simulink model "modele_non_lineaire"  (R2021a)
settings: Solver=VariableStepAuto  StartTime=0.0  StopTime=tfin  RelTol=1e-3
values from neighbouring files (symbols this model uses):
  ae0 = 1.339300    (= 1.3393)    [bancEssaiConstantes.m]
  ae1 = 3.57e+02    (= 357)    [bancEssaiConstantes.m]
  ae2 = 50.13    [bancEssaiConstantes.m]
  ae3 = 7.69e+05    (= 769000)    [bancEssaiConstantes.m]
  as0 = 0.0587    [bancEssaiConstantes.m]
  as1 = 22.606    [bancEssaiConstantes.m]
  as2 = 7.4466e+02    (= 744.66)    [bancEssaiConstantes.m]
  as3 = 2.458e+05    (= 245800)    [bancEssaiConstantes.m]
  be1 = 13.029359254409743    (= 13.0293592544)    [bancEssaiConstantes.m]
  g = 9.81    [bancEssaiConstantes.m]
  Jx = 1169e-06    (= 0.001169)    [bancEssaiConstantes.m]
  Jy = Jx    (= 0.001169)    [bancEssaiConstantes.m]
  LA = LL    (= 0.115)    [bancEssaiConstantes.m]
  LB = LL    (= 0.115)    [bancEssaiConstantes.m]
  LC = LL    (= 0.115)    [bancEssaiConstantes.m]
  mP = 425e-03    (= 0.425)    [bancEssaiConstantes.m]
  mSeff = mS+JS/rS^2    (= 0.0112)    [bancEssaiConstantes.m]
  mSg = mS*g    (= 0.07848)    [bancEssaiConstantes.m]
  RA = RR    (= 3.6)    [bancEssaiConstantes.m]
  RB = RR    (= 3.6)    [bancEssaiConstantes.m]
  RC = RR    (= 3.6)    [bancEssaiConstantes.m]
  XA = +rABC    (= 0.0952)    [bancEssaiConstantes.m]
  XB = -rABC*sind(30)    [bancEssaiConstantes.m]
  XC = -rABC*sind(30)    [bancEssaiConstantes.m]
  XD = +rDEF*sind(30)    [bancEssaiConstantes.m]
  XE = -rDEF    (= -0.08)    [bancEssaiConstantes.m]
  XF = +rDEF*sind(30)    [bancEssaiConstantes.m]
  YA = 0.0    (= 0)    [bancEssaiConstantes.m]
  YB = +rABC*cosd(30)    [bancEssaiConstantes.m]
  YC = -rABC*cosd(30)    [bancEssaiConstantes.m]
  YD = +rDEF*cosd(30)    [bancEssaiConstantes.m]
  YE = 0.0    (= 0)    [bancEssaiConstantes.m]
  YF = -rDEF*cosd(30)    [bancEssaiConstantes.m]
settings Model: Creator=royv2608  LastModifiedBy=User
settings SolverCC: AlgebraicLoopSolver=LineSearch

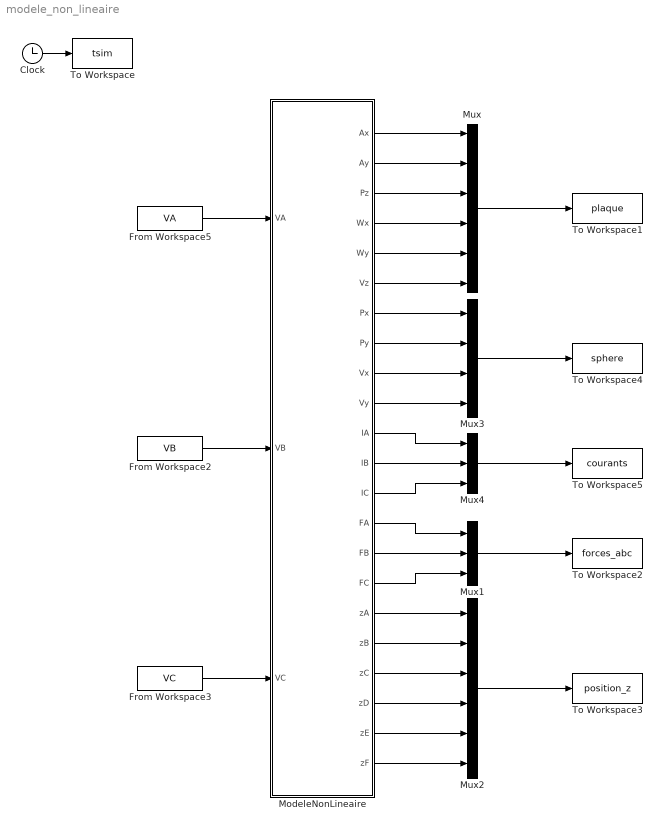
== system modele_non_lineaire ==
  Clock : Clock
  From Workspace2 : FromWorkspace  VariableName=VB  Interpolate=off  OutputAfterFinalValue=Holding final value
  From Workspace3 : FromWorkspace  VariableName=VC  Interpolate=off  OutputAfterFinalValue=Holding final value
  From Workspace5 : FromWorkspace  VariableName=VA  Interpolate=off  OutputAfterFinalValue=Holding final value
  ModeleNonLineaire : Subsystem
  Mux : Mux  Inputs=6
  Mux1 : Mux  Inputs=3
  Mux2 : Mux  Inputs=6
  Mux3 : Mux
  Mux4 : Mux  Inputs=3
  To Workspace : ToWorkspace  VariableName=tsim  SampleTime=-1
  To Workspace1 : ToWorkspace  VariableName=plaque  SampleTime=-1
  To Workspace2 : ToWorkspace  VariableName=forces_abc  SampleTime=-1
  To Workspace3 : ToWorkspace  VariableName=position_z  SampleTime=-1
  To Workspace4 : ToWorkspace  VariableName=sphere  SampleTime=-1
  To Workspace5 : ToWorkspace  VariableName=courants  SampleTime=-1
  wires:
  Clock/1 -> To Workspace/1
  Mux/1 -> To Workspace1/1
  From Workspace5/1 -> ModeleNonLineaire/1(VA)
  From Workspace3/1 -> ModeleNonLineaire/3(VC)
  ModeleNonLineaire/1(Ax) -> Mux/1
  ModeleNonLineaire/2(Ay) -> Mux/2
  ModeleNonLineaire/3(Pz) -> Mux/3
  ModeleNonLineaire/4(Wx) -> Mux/4
  ModeleNonLineaire/5(Wy) -> Mux/5
  ModeleNonLineaire/6(Vz) -> Mux/6
  ModeleNonLineaire/11(IA) -> Mux4/1
  ModeleNonLineaire/12(IB) -> Mux4/2
  ModeleNonLineaire/13(IC) -> Mux4/3
  ModeleNonLineaire/14(FA) -> Mux1/1
  ModeleNonLineaire/15(FB) -> Mux1/2
  ModeleNonLineaire/16(FC) -> Mux1/3
  Mux1/1 -> To Workspace2/1
  ModeleNonLineaire/17(zA) -> Mux2/1
  ModeleNonLineaire/19(zC) -> Mux2/3
  ModeleNonLineaire/18(zB) -> Mux2/2
  Mux2/1 -> To Workspace3/1
  From Workspace2/1 -> ModeleNonLineaire/2(VB)
  ModeleNonLineaire/20(zD) -> Mux2/4
  ModeleNonLineaire/21(zE) -> Mux2/5
  ModeleNonLineaire/22(zF) -> Mux2/6
  Mux3/1 -> To Workspace4/1
  ModeleNonLineaire/7(Px) -> Mux3/1
  ModeleNonLineaire/8(Py) -> Mux3/2
  ModeleNonLineaire/9(Vx) -> Mux3/3
  ModeleNonLineaire/10(Vy) -> Mux3/4
  Mux4/1 -> To Workspace5/1

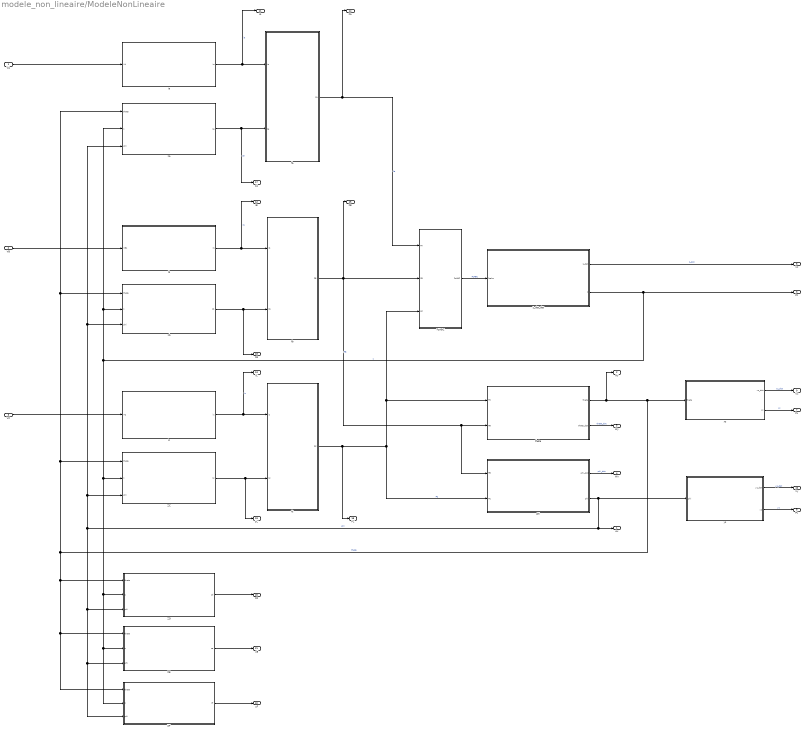
== system modele_non_lineaire/ModeleNonLineaire ==
  VA : Inport
  VB : Inport  Port=2
  VC : Inport  Port=3
  FzABC : Subsystem
  ZC : Subsystem
  ZD : Subsystem
  ZE : Subsystem
  ZF : Subsystem
  fa : Subsystem
  fb : Subsystem
  fc : Subsystem
  ia : Subsystem
  ib : Subsystem
  ic : Subsystem
  phi : Subsystem
  theta : Subsystem
  xs : Subsystem
  ys : Subsystem
  z_dot_dot : Subsystem
  za : Subsystem
  zb : Subsystem
  Ax : Outport
  Ay : Outport  Port=2
  Pz : Outport  Port=3
  Wx : Outport  Port=4
  Wy : Outport  Port=5
  Vz : Outport  Port=6
  Px : Outport  Port=7
  Py : Outport  Port=8
  Vx : Outport  Port=9
  Vy : Outport  Port=10
  IA : Outport  Port=11
  IB : Outport  Port=12
  IC : Outport  Port=13
  FA : Outport  Port=14
  FB : Outport  Port=15
  FC : Outport  Port=16
  zA : Outport  Port=17
  zB : Outport  Port=18
  zC : Outport  Port=19
  zD : Outport  Port=20
  zE : Outport  Port=21
  zF : Outport  Port=22
  wires:
  ia/1(ia) -> fa/1(ia), IA/1  "ia"
  ic/1(ic) -> IC/1, fc/1(ic)  "ic"
  phi/2(phi) -> ys/1(phi), Ax/1, za/3(phi), zb/3(phi), ZC/3(phi), ZD/3(phi), ZF/3(phi), ZE/3(phi)  "phi"
  theta/1(theta) -> xs/1(theta), ZD/1(theta), ZF/1(theta), ZE/1(theta), za/1(theta), zb/1(theta), ZC/1(theta), Ay/1  "theta"
  fa/1(FA) -> FzABC/1(FA), FA/1  "fa"
  fb/1(FB) -> FzABC/2(FB), phi/1(FB), theta/2(FB), FB/1  "FB"
  fc/1(FC) -> FC/1, phi/2(FC), FzABC/3(FC), theta/1(FC)  "FC"
  ZC/1(zc) -> zC/1, fc/2(zc)
  zb/1(zb) -> zB/1, fb/2(zb)
  ib/1(ib) -> fb/1(ib), IB/1  "ib"
  FzABC/1(FzABC) -> z_dot_dot/1(fzabc)  "FzABC"
  za/1(za) -> zA/1, fa/2(za)  "za"
  theta/2(theta_dot) -> Wy/1  "theta_dot"
  xs/1(xs_dot) -> Vx/1  "xs_dot"
  z_dot_dot/2(z) -> za/2(z), zb/2(z), ZD/2(z), ZF/2(z), ZE/2(z), ZC/2(z), Pz/1  "z"
  phi/1(phi_dot) -> Wx/1  "phi_dot"
  ys/2(ys) -> Py/1  "ys"
  VB/1 -> ib/1(VB1)
  z_dot_dot/1(z_dot) -> Vz/1  "z_dot"
  xs/2(xs) -> Px/1  "xs"
  ys/1(ys_dot) -> Vy/1  "ys_dot"
  VA/1 -> ia/1(VA)
  VC/1 -> ic/1(VC)
  ZD/1(zd) -> zD/1
  ZF/1(zf) -> zF/1
  ZE/1(ze) -> zE/1

== system modele_non_lineaire/ModeleNonLineaire/FzABC ==
  FA : Inport
  FB : Inport  Port=2
  FC : Inport  Port=3
  Sum of Elements : Sum  Inputs=---  CollapseDim=3
  FzABC : Outport
  wires:
  FC/1 -> Sum of Elements/3
  Sum of Elements/1 -> FzABC/1  "FzABC"
  FA/1 -> Sum of Elements/1
  FB/1 -> Sum of Elements/2

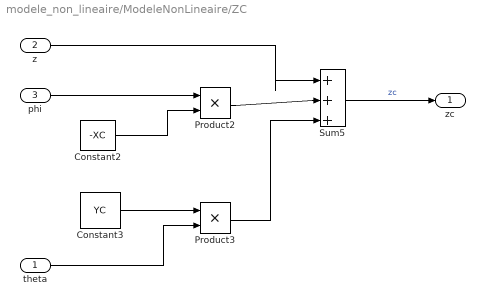
== system modele_non_lineaire/ModeleNonLineaire/ZC ==
  theta : Inport
  z : Inport  Port=2
  phi : Inport  Port=3
  Constant2 : Constant  Value=-XC
  Constant3 : Constant  Value=YC
  Product2 : Product
  Product3 : Product
  Sum5 : Sum  Inputs=|+++
  zc : Outport
  wires:
  Constant2/1 -> Product2/2
  z/1 -> Sum5/1
  theta/1 -> Product3/2
  Constant3/1 -> Product3/1
  phi/1 -> Product2/1
  Product3/1 -> Sum5/3
  Sum5/1 -> zc/1  "zc"
  Product2/1 -> Sum5/2

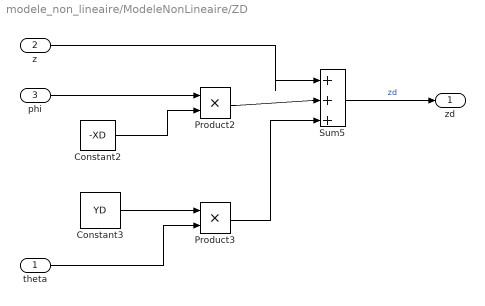
== system modele_non_lineaire/ModeleNonLineaire/ZD ==
  theta : Inport
  z : Inport  Port=2
  phi : Inport  Port=3
  Constant2 : Constant  Value=-XD
  Constant3 : Constant  Value=YD
  Product2 : Product
  Product3 : Product
  Sum5 : Sum  Inputs=|+++
  zd : Outport
  wires:
  Product2/1 -> Sum5/2
  Constant3/1 -> Product3/1
  Constant2/1 -> Product2/2
  phi/1 -> Product2/1
  z/1 -> Sum5/1
  Product3/1 -> Sum5/3
  theta/1 -> Product3/2
  Sum5/1 -> zd/1  "zd"

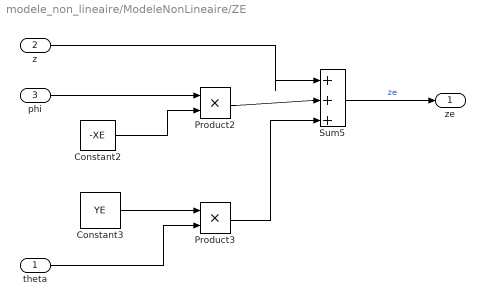
== system modele_non_lineaire/ModeleNonLineaire/ZE ==
  theta : Inport
  z : Inport  Port=2
  phi : Inport  Port=3
  Constant2 : Constant  Value=-XE
  Constant3 : Constant  Value=YE
  Product2 : Product
  Product3 : Product
  Sum5 : Sum  Inputs=|+++
  ze : Outport
  wires:
  Product2/1 -> Sum5/2
  Constant3/1 -> Product3/1
  Constant2/1 -> Product2/2
  phi/1 -> Product2/1
  z/1 -> Sum5/1
  Product3/1 -> Sum5/3
  theta/1 -> Product3/2
  Sum5/1 -> ze/1  "ze"

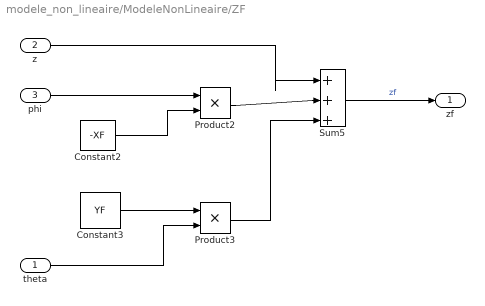
== system modele_non_lineaire/ModeleNonLineaire/ZF ==
  theta : Inport
  z : Inport  Port=2
  phi : Inport  Port=3
  Constant2 : Constant  Value=-XF
  Constant3 : Constant  Value=YF
  Product2 : Product
  Product3 : Product
  Sum5 : Sum  Inputs=|+++
  zf : Outport
  wires:
  Product2/1 -> Sum5/2
  Constant3/1 -> Product3/1
  Constant2/1 -> Product2/2
  phi/1 -> Product2/1
  z/1 -> Sum5/1
  Product3/1 -> Sum5/3
  theta/1 -> Product3/2
  Sum5/1 -> zf/1  "zf"

== system modele_non_lineaire/ModeleNonLineaire/fa ==
  ia : Inport
  za : Inport  Port=2
  fa : Subsystem
  FA : Outport
  wires:
  za/1 -> fa/2(za)
  ia/1 -> fa/1(ia)
  fa/1(FA) -> FA/1

== system modele_non_lineaire/ModeleNonLineaire/fb ==
  ib : Inport
  zb : Inport  Port=2
  FB_num : Subsystem
  FB : Outport
  wires:
  zb/1 -> FB_num/2(zb)
  ib/1 -> FB_num/1(ib)
  FB_num/1(FB) -> FB/1

== system modele_non_lineaire/ModeleNonLineaire/fc ==
  ic : Inport
  zc : Inport  Port=2
  fc : Subsystem
  FC : Outport
  wires:
  zc/1 -> fc/2(zc)
  ic/1 -> fc/1(ic)
  fc/1(FC) -> FC/1

== system modele_non_lineaire/ModeleNonLineaire/ia ==
  VA : Inport
  Gain : Gain  Gain=-RA/LA
  Gain1 : Gain  Gain=1/LA
  Integrator : Integrator
  Sum : Sum  Inputs=|++
  ia : Outport
  wires:
  Sum/1 -> Integrator/1  "ia_dot"
  Integrator/1 -> ia/1, Gain/1  "ia"
  Gain1/1 -> Sum/2
  Gain/1 -> Sum/1
  VA/1 -> Gain1/1

== system modele_non_lineaire/ModeleNonLineaire/ib ==
  VB1 : Inport
  Gain2 : Gain  Gain=-RB/LB
  Gain3 : Gain  Gain=1/LB
  Integrator1 : Integrator
  Sum1 : Sum  Inputs=|++
  ib : Outport
  wires:
  Sum1/1 -> Integrator1/1  "ib_dot"
  VB1/1 -> Gain3/1
  Integrator1/1 -> ib/1, Gain2/1  "ib"
  Gain2/1 -> Sum1/1
  Gain3/1 -> Sum1/2

== system modele_non_lineaire/ModeleNonLineaire/ic ==
  VC : Inport
  Gain4 : Gain  Gain=-RC/LC
  Gain5 : Gain  Gain=1/LC
  Integrator2 : Integrator
  Sum2 : Sum  Inputs=|++
  ic : Outport
  wires:
  Integrator2/1 -> ic/1, Gain4/1  "ic"
  Gain5/1 -> Sum2/2
  Gain4/1 -> Sum2/1
  Sum2/1 -> Integrator2/1  "ic_dot"
  VC/1 -> Gain5/1

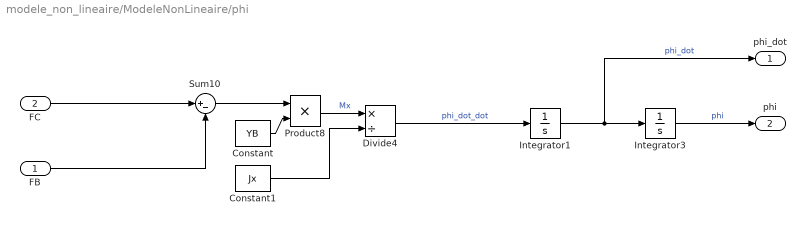
== system modele_non_lineaire/ModeleNonLineaire/phi ==
  FB : Inport
  FC : Inport  Port=2
  Constant : Constant  Value=YB
  Constant1 : Constant  Value=Jx
  Divide4 : Product  Inputs=*/
  Integrator1 : Integrator
  Integrator3 : Integrator
  Product8 : Product
  Sum10 : Sum  Inputs=|+-
  phi_dot : Outport
  phi : Outport  Port=2
  wires:
  Sum10/1 -> Product8/1
  Integrator3/1 -> phi/1  "phi"
  Product8/1 -> Divide4/1  "Mx"
  Constant/1 -> Product8/2
  Constant1/1 -> Divide4/2
  Integrator1/1 -> phi_dot/1, Integrator3/1  "phi_dot"
  Divide4/1 -> Integrator1/1  "phi_dot_dot"
  FC/1 -> Sum10/1
  FB/1 -> Sum10/2

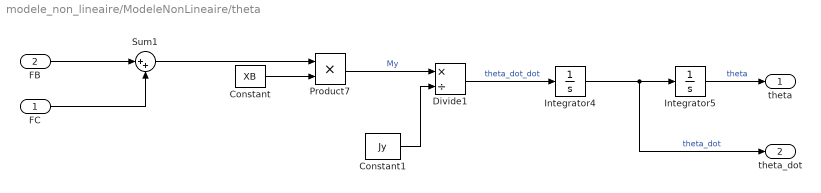
== system modele_non_lineaire/ModeleNonLineaire/theta ==
  FC : Inport
  FB : Inport  Port=2
  Constant : Constant  Value=XB
  Constant1 : Constant  Value=Jy
  Divide1 : Product  Inputs=*/
  Integrator4 : Integrator
  Integrator5 : Integrator
  Product7 : Product
  Sum1 : Sum  Inputs=|++
  theta : Outport
  theta_dot : Outport  Port=2
  wires:
  FB/1 -> Sum1/1
  FC/1 -> Sum1/2
  Constant1/1 -> Divide1/2
  Sum1/1 -> Product7/1
  Integrator4/1 -> theta_dot/1, Integrator5/1  "theta_dot"
  Product7/1 -> Divide1/1  "My"
  Constant/1 -> Product7/2
  Divide1/1 -> Integrator4/1  "theta_dot_dot"
  Integrator5/1 -> theta/1  "theta"

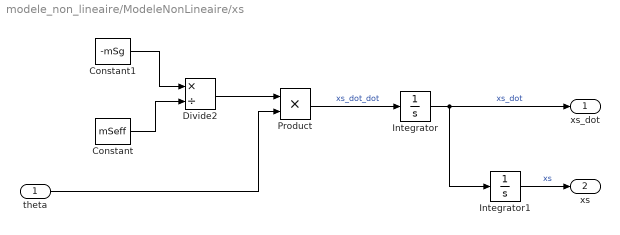
== system modele_non_lineaire/ModeleNonLineaire/xs ==
  theta : Inport
  Constant : Constant  Value=mSeff
  Constant1 : Constant  Value=-mSg
  Divide2 : Product  Inputs=*/
  Integrator : Integrator
  Integrator1 : Integrator
  Product : Product
  xs_dot : Outport
  xs : Outport  Port=2
  wires:
  Constant/1 -> Divide2/2
  Constant1/1 -> Divide2/1
  Divide2/1 -> Product/1
  theta/1 -> Product/2
  Product/1 -> Integrator/1  "xs_dot_dot"
  Integrator/1 -> Integrator1/1, xs_dot/1  "xs_dot"
  Integrator1/1 -> xs/1  "xs"

== system modele_non_lineaire/ModeleNonLineaire/ys ==
  phi : Inport
  Constant : Constant  Value=mSeff
  Constant1 : Constant  Value=mSg
  Divide1 : Product  Inputs=*/
  Integrator : Integrator
  Integrator1 : Integrator
  Product1 : Product
  ys_dot : Outport
  ys : Outport  Port=2
  wires:
  Constant/1 -> Divide1/2
  Divide1/1 -> Product1/1
  Constant1/1 -> Divide1/1
  phi/1 -> Product1/2
  Product1/1 -> Integrator/1  "ys_dot_dot"
  Integrator/1 -> Integrator1/1, ys_dot/1  "ys_dot"
  Integrator1/1 -> ys/1  "ys"

== system modele_non_lineaire/ModeleNonLineaire/z_dot_dot ==
  fzabc : Inport
  Constant1 : Constant  Value=mP
  Constant2 : Constant  Value=g
  Divide3 : Product  Inputs=*/
  Integrator : Integrator
  Integrator1 : Integrator
  Sum9 : Sum  Inputs=|++
  z_dot : Outport
  z : Outport  Port=2
  wires:
  Constant1/1 -> Divide3/2
  Constant2/1 -> Sum9/2
  Divide3/1 -> Sum9/1  "FB"
  fzabc/1 -> Divide3/1
  Sum9/1 -> Integrator/1  "z_dot_dot"
  Integrator/1 -> Integrator1/1, z_dot/1  "z_dot"
  Integrator1/1 -> z/1  "z"

== system modele_non_lineaire/ModeleNonLineaire/za ==
  theta : Inport
  z : Inport  Port=2
  phi : Inport  Port=3
  Constant1 : Constant  Value=-XA
  Constant2 : Constant  Value=YA
  Product2 : Product
  Product3 : Product
  Sum5 : Sum  Inputs=|+++
  za : Outport
  wires:
  z/1 -> Sum5/1
  Product3/1 -> Sum5/3
  Constant2/1 -> Product3/1
  Constant1/1 -> Product2/2
  Product2/1 -> Sum5/2
  Sum5/1 -> za/1  "za"
  theta/1 -> Product3/2
  phi/1 -> Product2/1

== system modele_non_lineaire/ModeleNonLineaire/zb ==
  theta : Inport
  z : Inport  Port=2
  phi : Inport  Port=3
  Constant : Constant  Value=-XB
  Constant1 : Constant  Value=YB
  Product2 : Product
  Product3 : Product
  Sum5 : Sum  Inputs=|+++
  zb : Outport
  wires:
  Constant1/1 -> Product3/1
  Constant/1 -> Product2/2
  Product3/1 -> Sum5/3
  Product2/1 -> Sum5/2
  theta/1 -> Product3/2
  Sum5/1 -> zb/1  "zb"
  phi/1 -> Product2/1
  z/1 -> Sum5/1

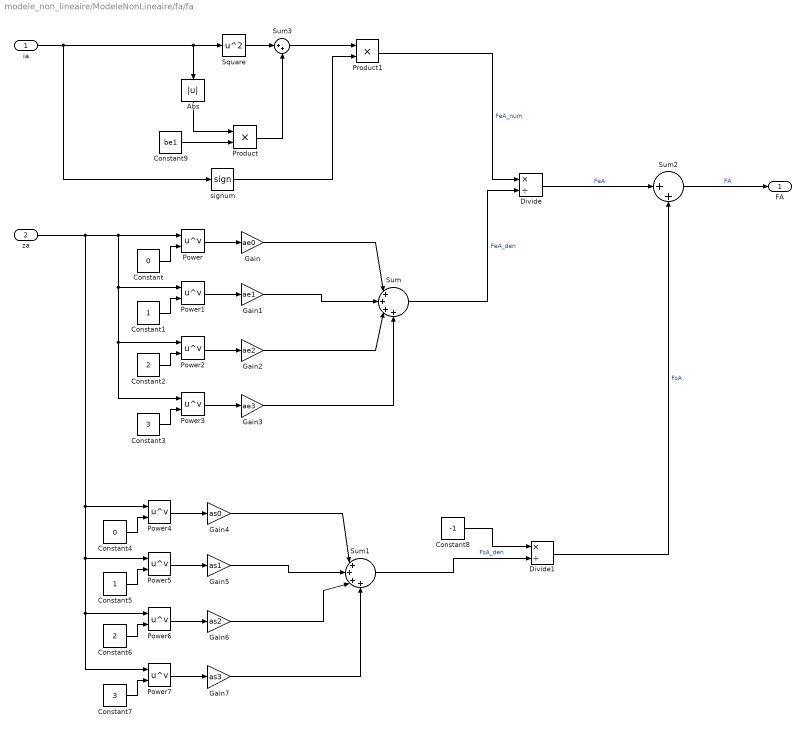
== system modele_non_lineaire/ModeleNonLineaire/fa/fa ==
  ia : Inport
  za : Inport  Port=2
  Abs : Abs
  Constant : Constant  Value=0
  Constant1 : Constant
  Constant2 : Constant  Value=2
  Constant3 : Constant  Value=3
  Constant4 : Constant  Value=0
  Constant5 : Constant
  Constant6 : Constant  Value=2
  Constant7 : Constant  Value=3
  Constant8 : Constant  Value=-1
  Constant9 : Constant  Value=be1
  Divide : Product  Inputs=*/
  Divide1 : Product  Inputs=*/
  Gain : Gain  Gain=ae0
  Gain1 : Gain  Gain=ae1
  Gain2 : Gain  Gain=ae2
  Gain3 : Gain  Gain=ae3
  Gain4 : Gain  Gain=as0
  Gain5 : Gain  Gain=as1
  Gain6 : Gain  Gain=as2
  Gain7 : Gain  Gain=as3
  Power{,1..7} (8 alike) : Math  Operator=pow  SaturateOnIntegerOverflow=on
  Product : Product
  Product1 : Product
  Square : Math  Operator=square  SaturateOnIntegerOverflow=on
  Sum : Sum  Inputs=|++++
  Sum1 : Sum  Inputs=|++++
  Sum2 : Sum  Inputs=|++
  Sum3 : Sum  Inputs=|++
  signum : Signum
  FA : Outport
  wires:
  Sum3/1 -> Product1/1
  signum/1 -> Product1/2
  Abs/1 -> Product/1
  ia/1 -> signum/1, Square/1, Abs/1
  Product/1 -> Sum3/2
  Square/1 -> Sum3/1
  Constant9/1 -> Product/2
  Product1/1 -> Divide/1  "FeA_num"
  Sum/1 -> Divide/2  "FeA_den"
  Power/1 -> Gain/1
  Gain2/1 -> Sum/3
  Power1/1 -> Gain1/1
  Gain3/1 -> Sum/4
  Power2/1 -> Gain2/1
  Gain1/1 -> Sum/2
  Gain/1 -> Sum/1
  Power3/1 -> Gain3/1
  Constant2/1 -> Power2/2
  Constant/1 -> Power/2
  Constant3/1 -> Power3/2
  Constant1/1 -> Power1/2
  Divide/1 -> Sum2/1  "FeA"
  Sum1/1 -> Divide1/2  "FsA_den"
  Power4/1 -> Gain4/1
  Gain6/1 -> Sum1/3
  Power5/1 -> Gain5/1
  Gain7/1 -> Sum1/4
  Power6/1 -> Gain6/1
  Gain5/1 -> Sum1/2
  Gain4/1 -> Sum1/1
  Power7/1 -> Gain7/1
  za/1 -> Power7/1, Power6/1, Power5/1, Power4/1, Power3/1, Power2/1, Power1/1, Power/1
  Constant6/1 -> Power6/2
  Constant4/1 -> Power4/2
  Constant7/1 -> Power7/2
  Constant5/1 -> Power5/2
  Constant8/1 -> Divide1/1
  Divide1/1 -> Sum2/2  "FsA"
  Sum2/1 -> FA/1  "FA"

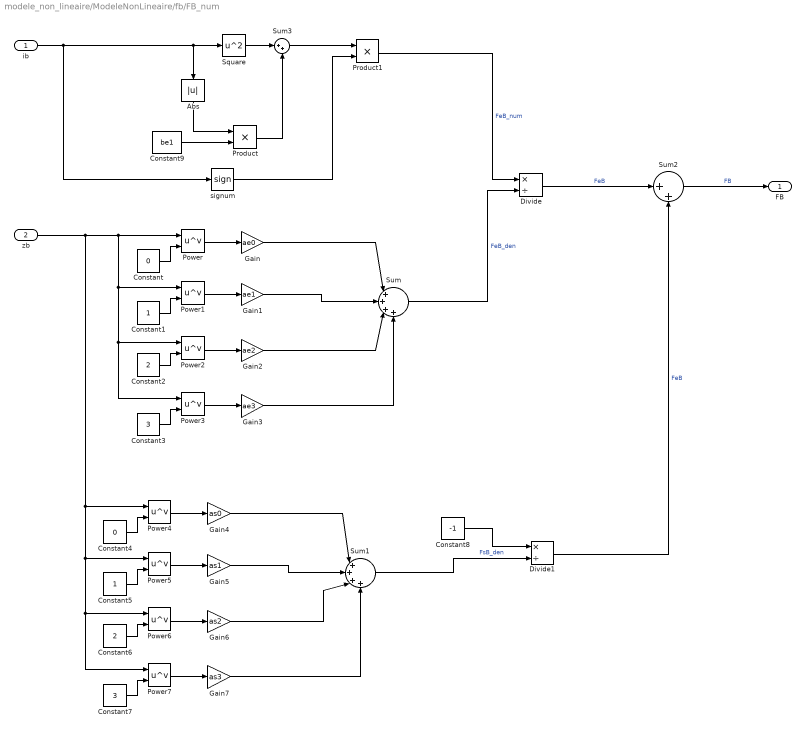
== system modele_non_lineaire/ModeleNonLineaire/fb/FB_num ==
  ib : Inport
  zb : Inport  Port=2
  Abs : Abs
  Constant : Constant  Value=0
  Constant1 : Constant
  Constant2 : Constant  Value=2
  Constant3 : Constant  Value=3
  Constant4 : Constant  Value=0
  Constant5 : Constant
  Constant6 : Constant  Value=2
  Constant7 : Constant  Value=3
  Constant8 : Constant  Value=-1
  Constant9 : Constant  Value=be1
  Divide : Product  Inputs=*/
  Divide1 : Product  Inputs=*/
  Gain : Gain  Gain=ae0
  Gain1 : Gain  Gain=ae1
  Gain2 : Gain  Gain=ae2
  Gain3 : Gain  Gain=ae3
  Gain4 : Gain  Gain=as0
  Gain5 : Gain  Gain=as1
  Gain6 : Gain  Gain=as2
  Gain7 : Gain  Gain=as3
  Power{,1..7} (8 alike) : Math  Operator=pow  SaturateOnIntegerOverflow=on
  Product : Product
  Product1 : Product
  Square : Math  Operator=square  SaturateOnIntegerOverflow=on
  Sum : Sum  Inputs=|++++
  Sum1 : Sum  Inputs=|++++
  Sum2 : Sum  Inputs=|++
  Sum3 : Sum  Inputs=|++
  signum : Signum
  FB : Outport
  wires:
  Sum3/1 -> Product1/1
  signum/1 -> Product1/2
  Abs/1 -> Product/1
  ib/1 -> signum/1, Square/1, Abs/1
  Product/1 -> Sum3/2
  Square/1 -> Sum3/1
  Constant9/1 -> Product/2
  Product1/1 -> Divide/1  "FeB_num"
  Sum/1 -> Divide/2  "FeB_den"
  Power/1 -> Gain/1
  Gain2/1 -> Sum/3
  Power1/1 -> Gain1/1
  Gain3/1 -> Sum/4
  Power2/1 -> Gain2/1
  Gain1/1 -> Sum/2
  Gain/1 -> Sum/1
  Power3/1 -> Gain3/1
  Constant2/1 -> Power2/2
  Constant/1 -> Power/2
  Constant3/1 -> Power3/2
  Constant1/1 -> Power1/2
  Divide/1 -> Sum2/1  "FeB"
  Sum1/1 -> Divide1/2  "FsB_den"
  Power4/1 -> Gain4/1
  Gain6/1 -> Sum1/3
  Power5/1 -> Gain5/1
  Gain7/1 -> Sum1/4
  Power6/1 -> Gain6/1
  Gain5/1 -> Sum1/2
  Gain4/1 -> Sum1/1
  Power7/1 -> Gain7/1
  zb/1 -> Power7/1, Power6/1, Power5/1, Power4/1, Power3/1, Power2/1, Power1/1, Power/1
  Constant6/1 -> Power6/2
  Constant4/1 -> Power4/2
  Constant7/1 -> Power7/2
  Constant5/1 -> Power5/2
  Constant8/1 -> Divide1/1
  Divide1/1 -> Sum2/2  "FeB"
  Sum2/1 -> FB/1  "FB"

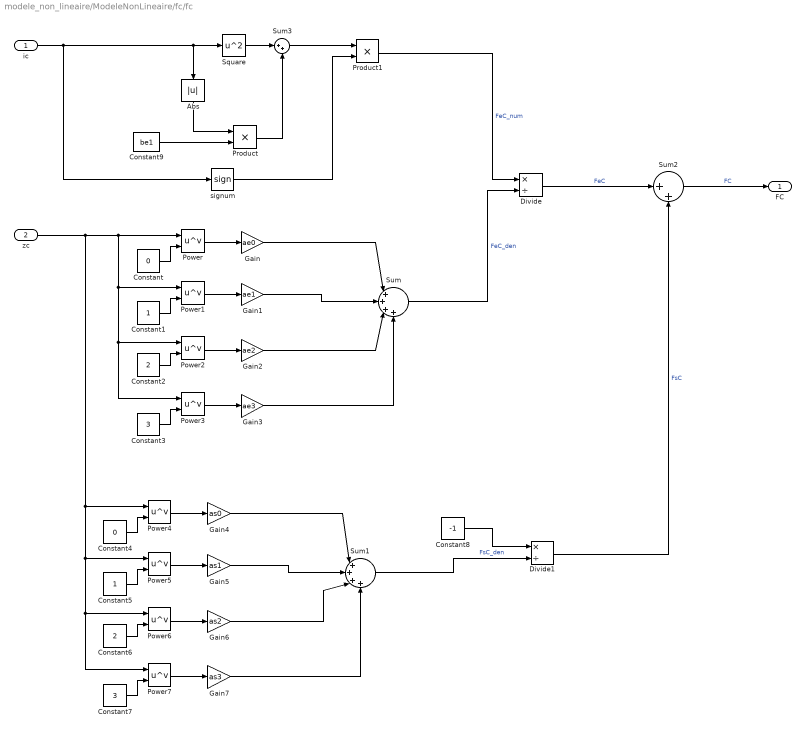
== system modele_non_lineaire/ModeleNonLineaire/fc/fc ==
  ic : Inport
  zc : Inport  Port=2
  Abs : Abs
  Constant : Constant  Value=0
  Constant1 : Constant
  Constant2 : Constant  Value=2
  Constant3 : Constant  Value=3
  Constant4 : Constant  Value=0
  Constant5 : Constant
  Constant6 : Constant  Value=2
  Constant7 : Constant  Value=3
  Constant8 : Constant  Value=-1
  Constant9 : Constant  Value=be1
  Divide : Product  Inputs=*/
  Divide1 : Product  Inputs=*/
  Gain : Gain  Gain=ae0
  Gain1 : Gain  Gain=ae1
  Gain2 : Gain  Gain=ae2
  Gain3 : Gain  Gain=ae3
  Gain4 : Gain  Gain=as0
  Gain5 : Gain  Gain=as1
  Gain6 : Gain  Gain=as2
  Gain7 : Gain  Gain=as3
  Power{,1..7} (8 alike) : Math  Operator=pow  SaturateOnIntegerOverflow=on
  Product : Product
  Product1 : Product
  Square : Math  Operator=square  SaturateOnIntegerOverflow=on
  Sum : Sum  Inputs=|++++
  Sum1 : Sum  Inputs=|++++
  Sum2 : Sum  Inputs=|++
  Sum3 : Sum  Inputs=|++
  signum : Signum
  FC : Outport
  wires:
  Sum3/1 -> Product1/1
  signum/1 -> Product1/2
  Abs/1 -> Product/1
  ic/1 -> signum/1, Square/1, Abs/1
  Product/1 -> Sum3/2
  Square/1 -> Sum3/1
  Constant9/1 -> Product/2
  Product1/1 -> Divide/1  "FeC_num"
  Sum/1 -> Divide/2  "FeC_den"
  Power/1 -> Gain/1
  Gain2/1 -> Sum/3
  Power1/1 -> Gain1/1
  Gain3/1 -> Sum/4
  Power2/1 -> Gain2/1
  Gain1/1 -> Sum/2
  Gain/1 -> Sum/1
  Power3/1 -> Gain3/1
  Constant2/1 -> Power2/2
  Constant/1 -> Power/2
  Constant3/1 -> Power3/2
  Constant1/1 -> Power1/2
  Divide/1 -> Sum2/1  "FeC"
  Sum1/1 -> Divide1/2  "FsC_den"
  Power4/1 -> Gain4/1
  Gain6/1 -> Sum1/3
  Power5/1 -> Gain5/1
  Gain7/1 -> Sum1/4
  Power6/1 -> Gain6/1
  Gain5/1 -> Sum1/2
  Gain4/1 -> Sum1/1
  Power7/1 -> Gain7/1
  zc/1 -> Power7/1, Power6/1, Power5/1, Power4/1, Power3/1, Power2/1, Power1/1, Power/1
  Constant6/1 -> Power6/2
  Constant4/1 -> Power4/2
  Constant7/1 -> Power7/2
  Constant5/1 -> Power5/2
  Constant8/1 -> Divide1/1
  Divide1/1 -> Sum2/2  "FsC"
  Sum2/1 -> FC/1  "FC"
